simulink model "mixed_"  (Simulink 7.0)
settings: Solver=ode45  SolverMode=SingleTasking  StartTime=0.0  StopTime=3  FixedStep=.25  MaxStep=3  RelTol=1e-6
settings Model: Creator=dyblenko  LastModifiedBy=dyblenko

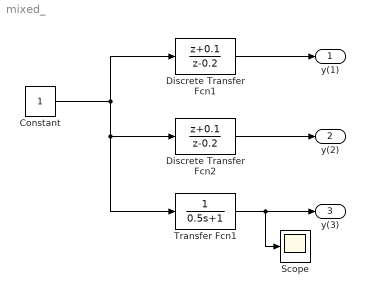
== system mixed_ ==
  Constant : Constant  OutDataType=sfix(16)  OutScaling=2^0
  Discrete Transfer Fcn1 : DiscreteTransferFcn  Numerator=[1 0.1]  Denominator=[1 -0.2]  SampleTime=0.75
  Discrete Transfer Fcn2 : DiscreteTransferFcn  Numerator=[1 0.1]  Denominator=[1 -0.2]  SampleTime=0.5
  Scope : Scope
  Transfer Fcn1 : TransferFcn  Denominator=[0.5 1]
  y(1) : Outport  OutDataType=sfix(16)  OutScaling=2^0
  y(2) : Outport  Port=2  OutDataType=sfix(16)  OutScaling=2^0
  y(3) : Outport  Port=3  OutDataType=sfix(16)  OutScaling=2^0
  wires:
  Constant/1 -> Discrete Transfer Fcn1/1, Discrete Transfer Fcn2/1, Transfer Fcn1/1
  Discrete Transfer Fcn1/1 -> y(1)/1
  Discrete Transfer Fcn2/1 -> y(2)/1
  Transfer Fcn1/1 -> y(3)/1, Scope/1
